simulink model "CL_SC"  (R2024a)
settings: Solver=FixedStepDiscrete  StartTime=0.0  StopTime=inf  FixedStep=Ts  RelTol=RelativeTolerance  EnableMultiTasking=on
undefined symbols (not defined in the file): DenZ, NumZ, Ts
libraries: c2837xDlib x1
settings Model: SimulationMode=external  ExtModeTrigDuration=8  Creator=Fernand  LastModifiedBy=cesar
settings DataIOCC: SaveFormat=StructureWithTime  ReturnWorkspaceOutputs=off  OutputSaveName=data_results  SignalLoggingName=DataResult
settings OptimizationCC: DefaultUnderspecifiedDataType=single  EnhancedBackFolding=on  PassReuseOutputArgsAs=Individual arguments  MaxStackSize=1024  OptimizeBlockOrder=speed  DifferentSizesBufferReuse=on  OptimizationCustomize=off  EfficientTunableParamExpr=on
settings DebuggingCC: ParameterTunabilityLossMsg=error
settings HardwareCC: ProdBitPerChar=16  ProdBitPerInt=16  ProdBitPerPointer=32  ProdBitPerSizeT=32  ProdBitPerPtrDiffT=32  ProdLargestAtomicInteger=Integer  ProdLargestAtomicFloat=None  ProdWordSize=16  ProdLongLongMode=on  ProdHWDeviceType=Texas Instruments->C2000  HardwareBoardFeatureSet=SoCBlockset
settings ModelReferenceCC: ModelReferenceNumInstancesAllowed=Single
settings SFSimCC: MATLABDynamicMemAlloc=off
settings RTWCC: Description=Embedded Coder  SystemTargetFile=ert.tlc  HardwareBoard=TI Delfino F28379D LaunchPad  TemplateMakefile=ert_default_tmf  Toolchain=Texas Instruments Code Composer Studio (C2000)  CodeProfilingSaveOptions=MetricsOnly  GPUComputeCapability=3.5
settings CodeAppCC: ForceParamTrailComments=on  IgnoreCustomStorageClasses=off  OperatorAnnotations=on  SimulinkDataObjDesc=on  SFDataObjDesc=on  InsertBlockDesc=on
settings ERTTargetCC: CodeReplacementLibrary=TI C28x  ExtMode=on  ExtModeTransport=4  ExtModeStaticAlloc=on  ExtModeAutomaticAllocSize=off  ExtModeStaticAllocSize=10000  ExtModeMexFile=ext_xcp  ExtModeMexArgs=1 6 5000000  ExtModeIntrfLevel=Level2 - Open

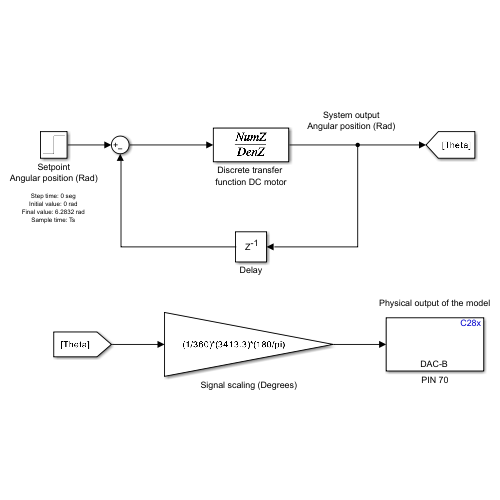
[thumbnail: Simulink's stored preview of the top-level diagram]
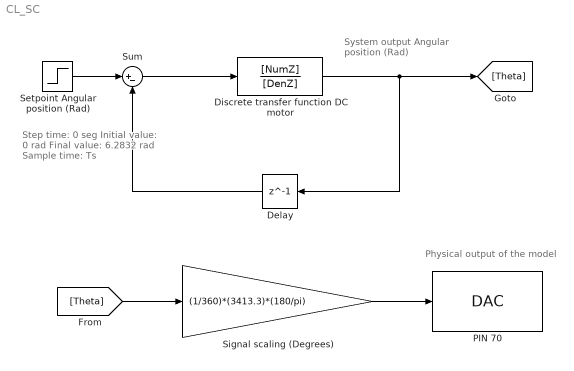
== system CL_SC ==
  note: Step time: 0 seg
      | Initial value: 0 rad
      | Final value: 6.2832 rad
      | Sample time: Ts
  note: System output
      | Angular position (Rad)
  note: Physical output of the model
  " Delay " : Delay  DelayLength=1  SampleTime=Ts
  Discrete transfer function DC motor : DiscreteTransferFcn  Numerator=[NumZ]  Denominator=[DenZ]  SampleTime=Ts
  PIN 70 : c2837xDlib/DAC  channel=B  saturate=on
  Setpoint Angular position (Rad) : Step  Time=0  After=2*pi  SampleTime=Ts
  Signal scaling (Degrees) : Gain  Gain=(1/360)*(3413.3)*(180/pi)  OutDataTypeStr=single
  Sum : Sum  Inputs=|+-
  wires:
  [Theta] -> Signal scaling (Degrees)/1
  Sum/1 -> Discrete transfer function DC motor/1
  " Delay "/1 -> Sum/2
  Setpoint Angular position (Rad)/1 -> Sum/1
  Discrete transfer function DC motor/1 -> " Delay "/1, [Theta]
  Signal scaling (Degrees)/1 -> PIN 70/1
